simulink model "Backhoe_Arm"  (R2014a)
settings: Solver=ode23t  StartTime=0.0  StopTime=10  MaxStep=0.01  RelTol=1e-3
PostLoadFcn:
  | warning off sm:compiler:state:UnsatisfiedDesiredTarget
  | warning off simscape:compiler:sli:init:SolverNotRecommended
  | warning off sm:sli:visualization:UnsupportedSimMode
  | warning off xPCTarget:sampleTime:sampleTimeInvariance
  | warning off Simulink:blocks:MatchingFromNotFound
model workspace (MAT data in the model file):
  cylinderGray = [0.6 0.6 0.6]
  darkOrange = [0.8 0.5 0]
  glassBlue = [0.2 0.2 1]
  gray = [0.3 0.3 0.3]
  orange = [0.8 0.65 0]
  pistonGray = [0.4 0.4 0.4]
  tireBlack = [0.1 0.1 0.1]
  wheelGray = [0.6 0.6 0.6]
  yellow = [0.8 0.8 0]
  rhoGlass = 2500
  rhoRubber = 1500
  rhoSteel = 7800
undefined symbols (not defined in the file): sigbuilder_block, X, Y, Z
libraries: sm_lib x78, Backhoe_Lib x12, nesl_utility x3
(part 1 of 3)
Description:
  | Copyright 2014 The MathWorks, Inc.
settings Model: ExtModeTrigDuration=3334  BufferReuse=off  Creator=smiller  LastModifiedBy=Olli
settings SolverCC: EnableConcurrentExecution=on
settings DataIOCC: LimitDataPoints=off  SignalLoggingSaveFormat=ModelDataLogs
settings OptimizationCC: BlockReduction=off  OptimizeBlockIOStorage=off  BufferReuse=off  GlobalBufferReuse=off  ExpressionFolding=off  ExpressionDepthLimit=2147483647  LocalBlockOutputs=off
settings DebuggingCC: UnderspecifiedInitializationDetection=Classic  SolverPrmCheckMsg=none  MultiTaskDSMMsg=warning  MultiTaskCondExecSysMsg=none  StateNameClashWarn=warning
settings HardwareCC: ProdIntDivRoundTo=Zero  ProdEndianess=LittleEndian  ProdHWDeviceType=Generic->32-bit x86 compatible
settings RTWCC: SystemTargetFile=slrt.tlc  TemplateMakefile=slrt_default_tmf  Description=Simulink Real-Time  ProcessScript=slrt_make_rtw_hook  IncludeERTFirstTime=on  RTWCompilerOptimization=On
settings SimulinkRealTimeCC: GeneratePreprocessorConditionals=Disable all  EnableShiftOperators=on  RL32LogBufSizeModifier=300000
settings SimscapeCC: ExplicitSolverDiagnosticOptions=none
settings SimMechanicsCC: WarnOnRedundantConstraints=off
settings ExplorerConfigSet: InternalSimMechanicsExplorerSettings="<ExplorerConfiguration><canonicalview>default</canonicalview><TilePanel><TileInfo><Tiles Columns=\"1\" Count=\"1\" Rows=\"1\"><Column Left=\"2\" Weight=\"1\"/><Column Left=\"525\"/><Row Top=\"2\" Weight=\"1\"/><Row Top=\"370\"/><Tile Height=\"1\" Width=\"1\" X=\"0\" Y=\"0\"/></Tiles></TileInfo><SceneInfo><SceneViewer><BGColor><R>0.60000002384185791</R><G>0.60000002384185791</G><B>0.60000002384185791</B></BGColor><Camera><Position><X>16.211716622846833</X><Y>-13.061299378004865</Y><Z>8.3540336197668257</Z></Position><Center><X>-0.88618319905958465</X><Y>-6.5797450383619722</Y><Z>3.3077110306737345</Z></Center><Up><X>-0.26232421756367919</X><Y>0.057951672533943753</Y><Z>0.96323808507041631</Z></Up><Left>-4.3797052145004276</Left><Right>4.3797052145004276</Right><Bottom>-5.0912822484970093</Bottom><Top>5.0912822484970093</Top></Camera></SceneViewer></SceneInfo></TilePanel></ExplorerConfiguration>"

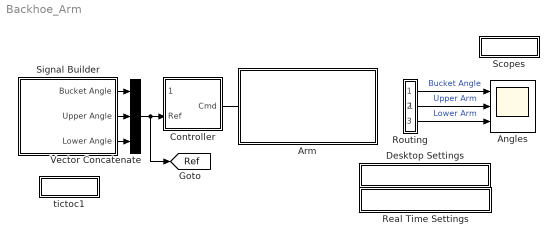
== system Backhoe_Arm ==
  Angles : Scope  NumInputPorts=3
      settings: TimeRange=60  YMin=-120~-20~-60  YMax=20~60~0
  Arm : Subsystem
      mask Display:
      | image(imread('Backhoe_Arm_IMAGE.JPG'));
      | port_label('input',1,'Cmd');
      | port_label('Output',1,'Meas');
  Controller : Subsystem
  Desktop Settings : Subsystem
      settings: OpenFcn=|
      | set_param(bdroot,'Solver','ODE23t','MaxStep','0.01','RelTol','1e-3','AbsTol','auto');
      | tvar_solverBlock = find_system(bdroot, 'SubClassName', 'solver');
      | 
      | for i=1:size(tvar_solverBlock,1)
      | 
      | set_param(char(tvar_solverBlock(i)), 'UseLocalSolver','off','DoFixedCost','off');
      | end
      | 
      | clear tvar_solverBlock
      mask Display: disp('Desktop Settings')
  Real Time Settings : Subsystem
      settings: OpenFcn=|
      | tvar_Nonlinear_Iterations = '2';
      | tvar_StepSize = '0.0004';                                                                                              %tvar_LocalSolver = 'NE_TRAPEZOIDAL_ADVANCER';
      | tvar_LocalSolver = 'NE_BACKWARD_EULER_ADVANCER';
      | set_param(bdroot,'Solver','ode1','FixedStep','auto');
      | tvar_solverBlock = find_system(bdroot, 'SubClassName', 'solver');
      | for i=1:size(tvar_solverBlock,1)
      | 
      | set_param(char(tvar_solverBlock(i)), 'UseLocalSolver','on','DoFixedCost','on','MaxNonlinIter',tvar_Nonlinear_Iterations,'LocalSolverChoice',tvar_LocalSolver,'LocalSolverSampleTime',tvar_StepSize);
      | end
      | clear tvar_Nonlinear_Iterations tvar_StepSize tvar_LocalSolver tvar_solverBlock
      mask Display: disp('Real Time Settings')
  Routing : Subsystem
  Scopes : Subsystem
  Signal Builder : Subsystem  Tag=STV Subsys  LoadFcn=sigbuilder_block('load');  StartFcn=sigbuilder_block('start');  StopFcn=sigbuilder_block('stop');  ClipboardFcn=sigbuilder_block('clipboard');  mask(Sigbuilder block){}
      mask help: Simulink:masks:SigbuilderBlock_MD
      mask init:
      | if ~strcmp(get_param(bdroot(gcbh),'SimulationStatus'),'stopped') tuvar = sigbuilder_block('maskInit'); end
      settings: CopyFcn=sigbuilder_block('copy');  DeleteFcn=sigbuilder_block('delete');  ModelCloseFcn=sigbuilder_block('modelClose');  PreSaveFcn=sigbuilder_block('preSave');  PauseFcn=sigbuilder_block('pause');  ContinueFcn=sigbuilder_block('continue');  NameChangeFcn=sigbuilder_block('namechange');  OpenFcn=sigbuilder_block('open',[5.58621 8.06897 624.414 412.759 ]);  CloseFcn=sigbuilder_block('close');
      mask Display: plot(0, 0, 100, 100,[2, 2, 32, 32, 2], [68, 8, 8, 68, 68],[32, 2], [38, 38], [32, 19, 2],[53, 60, 44], [32, 17, 17, 2],[16, 16, 31, 31]);txt = getActiveGroup(gcbh);text(2, 100, txt,'verticalAlignment', 'top');
  Vector Concatenate : Concatenate  NumInputs=3
  tictoc1 : Subsystem
      settings: OpenFcn=open('Backhoe_Demo_Script.html')
      mask Display: disp('Script')
  tag scope: Ref=global
  wires:
  Signal Builder/2(Upper Angle) -> Vector Concatenate/2
  Signal Builder/1(Bucket Angle) -> Vector Concatenate/1
  Signal Builder/3(Lower Angle) -> Vector Concatenate/3
  Vector Concatenate/1 -> [Ref], Controller/2(Ref)
  ? -> Controller/1(Meas), Routing/1(Meas)
  Controller/1(Cmd) -> ?
  Routing/2(UArm) -> Angles/2  "Upper Arm"
  Routing/3(LArm) -> Angles/3  "Lower Arm"
  Routing/1(Bucket) -> Angles/1  "Bucket Angle"

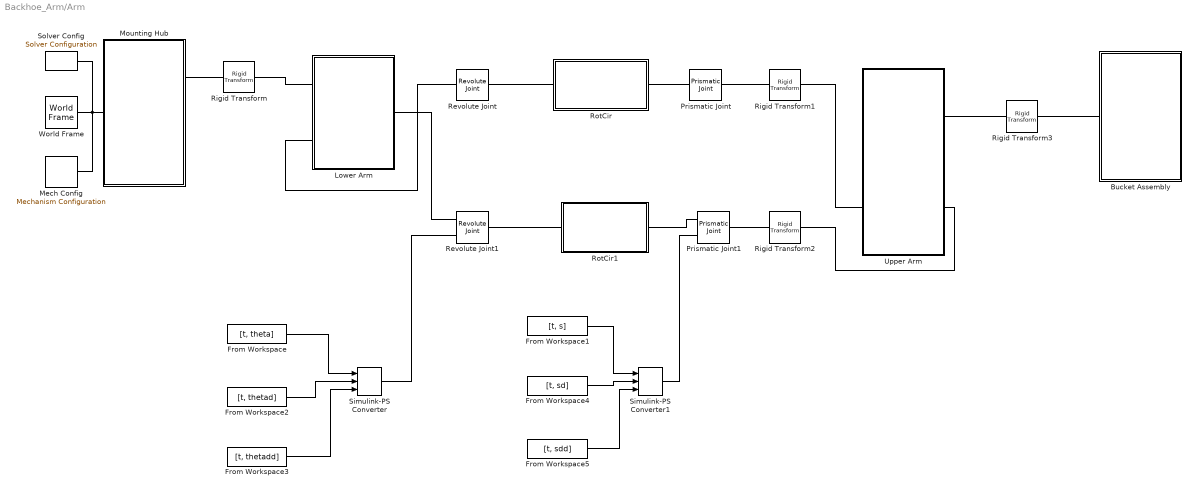
== system Backhoe_Arm/Arm ==
  Bucket Assembly : Subsystem
      mask Display:
      | image(imread('Backhoe_Arm_Bucket_Asy_IMAGE.JPG'));
      | port_label('lconn',1,'UAL');
      | port_label('lconn',2,'UAR');
      | port_label('lconn',3,'UA');
      | port_label('rconn',1,'TAct');
  From Workspace : FromWorkspace  VariableName=[t, theta]
  From Workspace1 : FromWorkspace  VariableName=[t, s]
  From Workspace2 : FromWorkspace  VariableName=[t, thetad]
  From Workspace3 : FromWorkspace  VariableName=[t, thetadd]
  From Workspace4 : FromWorkspace  VariableName=[t, sd]
  From Workspace5 : FromWorkspace  VariableName=[t, sdd]
  "Lower Arm " : Subsystem
      mask Display:
      | image(imread('Backhoe_Arm_Lower_IMAGE.JPG'));
      | port_label('lconn',1,'H');
      | port_label('lconn',2,'LAct');
      | port_label('rconn',1,'UA');
      | port_label('rconn',2,'RAct');
  Mech Config : sm_lib/Utilities/Mechanism Configuration  UniformGravity=Constant  GravityVector=[0 0 -9.81]  GravityUnits=m/s^2  LinearizationDelta=0.001  BlockFunction=simmechanics.library.utilities.mechanism_configuration
  Mounting Hub : Subsystem  mask(Mounting Hub){Hleft=1, Hright=2, Ltop=0.75, Lbottom=1.5, Tplate=0.3, Dplates=1.2, plateFillet=0.25, numPoints=15, L1=0.75, H1=0.25, RH1=0.075, L2=0.75, H2=1.75, RH2=0.075, L3=0.5, H3=0.5, Larm=0.8, Warm=0.5, Tarm=0.5, Tab=0.1, RH3=0.075, Dbracket=1.1, Lbracket=1.2, Wbracket=1.2, Tbracket=2, Hbracket=1, Rhole=0.1, Hhole=0.5, hubColor=orange, rho=rhoSteel}
      mask prompts: Hleft "Hleft [m]"; Hright "Hright [m]"; Ltop "Ltop [m]"; Lbottom "Lbottom [m]"; Tplate "Tplate [m]"; Dplates "Dplates [m]"; plateFillet "Plate Fillet Radius [m]"; numPoints "Fillet Point Resolution"; L1 "L1 [m]"; H1 "H1 [m]"; RH1 "RH1 [m]"; L2 "L2 [m]"; H2 "H2 [m]"; RH2 "RH2 [m]"; L3 "L3 [m]"; H3 "H3 [m]"; Larm "Larm [m]"; Warm "Warm [m]"; Tarm "Tarm [m]"; Tab "Tab [m]"; RH3 "RH3 [m]"; Dbracket "Dbracket [m]"; Lbracket "Lbracket [m]"; Wbracket "Wbracket [m]"; Tbracket "Tbracket [m]"; Hbracket "Hbracket [m]"; Rhole "Rhole [m]"; Hhole "Hhole [m]"; hubColor "Hub Color"; rho "Density [kg/m^3]"
      mask help:
      | Consists of the backhoe mounting hub assembly.
      |
      | This assembly connects to the Backhoe Arm assembly on the front end, and to the Mounting Base assembly on the rear and side.
      |
      | Attachment points are:
      | LH: Left base hydraulic actuator (piston Head).
      | RH: Right base hydraulic actuator (piston Head).
      | LC: Lower arm hydraulic actuator (Cylinder base).
      | LA: Lower Arm joint.
      | MB: Mounting Base joint.
      | All attachments are configured for Revolute Joints.
      |
      | Click on Help to view a schematic of the bracket, its configurable dimension parameters and attachment points (in red).
      mask init:
      | plateSection = [0              0     ; ...
      |                 Lbottom        0     ; ...
      |                 Lbottom        Hright; ...
      |                 (Lbottom-Ltop) Hright; ...
      |                 0              Hleft];
      | plateSection = Extr_Data_Round_Corners(plateSection,1:5,0.1,15);
      mask Help: web('Backhoe_Mountinghub.html');
      mask Display:
      | image(imread('Backhoe_Arm_Base_IMAGE.JPG'));
      | port_label('lconn',1,'B');
      | port_label('rconn',1,'LArm');
      | port_label('rconn',2,'LAct');
  Prismatic Joint : sm_lib/Joints/Prismatic Joint  SenseConstraintForce=off  SenseConstraintForceX=off  SenseConstraintForceY=off  SenseConstraintForceZ=off  SenseConstraintTorque=off  SenseConstraintTorqueX=off  SenseConstraintTorqueY=off  SenseConstraintTorqueZ=off  SenseTotalForce=off  SenseTotalForceX=off  SenseTotalForceY=off  SenseTotalForceZ=off  SenseTotalTorque=off  SenseTotalTorqueX=off  SenseTotalTorqueY=off  SenseTotalTorqueZ=off  CompositeWrenchDir=FollowerOnBase  CompositeWrenchFrame=BaseFrame  EquilibriumPosition=0  EquilibriumPositionUnits=m  SpringStiffness=0  SpringStiffnessUnits=N/m  DampingCoefficient=0  DampingCoefficientUnits=N/(m/s)  TorqueActuationMode=NoTorque  MotionActuationMode=ComputedMotion  SensePosition=off  SenseVelocity=off  SenseAcceleration=off  SenseTorqueForce=off  PositionTargetValue=0  PositionTargetValueUnits=m  PositionTargetSpecify=off  PositionTargetPriority=High  VelocityTargetValue=0.001  VelocityTargetValueUnits=m/s  VelocityTargetSpecify=on  VelocityTargetPriority=High  BlockFunction=simmechanics.library.joints.prismatic_joint
  Prismatic Joint1 : sm_lib/Joints/Prismatic Joint  SenseConstraintForce=off  SenseConstraintForceX=off  SenseConstraintForceY=off  SenseConstraintForceZ=off  SenseConstraintTorque=off  SenseConstraintTorqueX=off  SenseConstraintTorqueY=off  SenseConstraintTorqueZ=off  SenseTotalForce=off  SenseTotalForceX=off  SenseTotalForceY=off  SenseTotalForceZ=off  SenseTotalTorque=off  SenseTotalTorqueX=off  SenseTotalTorqueY=off  SenseTotalTorqueZ=off  CompositeWrenchDir=FollowerOnBase  CompositeWrenchFrame=BaseFrame  EquilibriumPosition=0  EquilibriumPositionUnits=m  SpringStiffness=0  SpringStiffnessUnits=N/m  DampingCoefficient=0  DampingCoefficientUnits=N/(m/s)  TorqueActuationMode=ComputedTorque  MotionActuationMode=InputMotion  SensePosition=off  SenseVelocity=off  SenseAcceleration=off  SenseTorqueForce=off  PositionTargetValue=0  PositionTargetValueUnits=m  PositionTargetSpecify=off  PositionTargetPriority=High  VelocityTargetValue=0.001  VelocityTargetValueUnits=m/s  VelocityTargetSpecify=on  VelocityTargetPriority=High  BlockFunction=simmechanics.library.joints.prismatic_joint
  Revolute Joint : sm_lib/Joints/Revolute Joint  SenseConstraintForce=off  SenseConstraintForceX=off  SenseConstraintForceY=off  SenseConstraintForceZ=off  SenseConstraintTorque=off  SenseConstraintTorqueX=off  SenseConstraintTorqueY=off  SenseConstraintTorqueZ=off  SenseTotalForce=off  SenseTotalForceX=off  SenseTotalForceY=off  SenseTotalForceZ=off  SenseTotalTorque=off  SenseTotalTorqueX=off  SenseTotalTorqueY=off  SenseTotalTorqueZ=off  CompositeWrenchDir=FollowerOnBase  CompositeWrenchFrame=BaseFrame  EquilibriumPosition=0  EquilibriumPositionUnits=deg  SpringStiffness=0  SpringStiffnessUnits=N*m/deg  DampingCoefficient=0  DampingCoefficientUnits=N*m/(deg/s)  TorqueActuationMode=NoTorque  MotionActuationMode=ComputedMotion  SensePosition=off  SenseVelocity=off  SenseAcceleration=off  SenseTorqueForce=off  PositionTargetValue=0  PositionTargetValueUnits=deg  PositionTargetSpecify=off  PositionTargetPriority=High  VelocityTargetValue=45  VelocityTargetValueUnits=deg/s  VelocityTargetSpecify=off  VelocityTargetPriority=High  BlockFunction=simmechanics.library.joints.revolute_joint
  Revolute Joint1 : sm_lib/Joints/Revolute Joint  SenseConstraintForce=off  SenseConstraintForceX=off  SenseConstraintForceY=off  SenseConstraintForceZ=off  SenseConstraintTorque=off  SenseConstraintTorqueX=off  SenseConstraintTorqueY=off  SenseConstraintTorqueZ=off  SenseTotalForce=off  SenseTotalForceX=off  SenseTotalForceY=off  SenseTotalForceZ=off  SenseTotalTorque=off  SenseTotalTorqueX=off  SenseTotalTorqueY=off  SenseTotalTorqueZ=off  CompositeWrenchDir=FollowerOnBase  CompositeWrenchFrame=BaseFrame  EquilibriumPosition=0  EquilibriumPositionUnits=deg  SpringStiffness=0  SpringStiffnessUnits=N*m/deg  DampingCoefficient=0  DampingCoefficientUnits=N*m/(deg/s)  TorqueActuationMode=ComputedTorque  MotionActuationMode=InputMotion  SensePosition=off  SenseVelocity=off  SenseAcceleration=off  SenseTorqueForce=off  PositionTargetValue=0  PositionTargetValueUnits=deg  PositionTargetSpecify=off  PositionTargetPriority=High  VelocityTargetValue=45  VelocityTargetValueUnits=deg/s  VelocityTargetSpecify=off  VelocityTargetPriority=High  BlockFunction=simmechanics.library.joints.revolute_joint
  Rigid Transform : sm_lib/Frames and Transforms/Rigid Transform  TranslationMethod=None  TranslationLengthUnit=m  TranslationStandardAxis=+Z  TranslationStandardOffset=0  TranslationCartesianOffset=[0 0 0]  TranslationROffset=0  TranslationROffsetUnits=m  TranslationZOffset=0  TranslationZOffsetUnits=m  TranslationThetaOffset=0  TranslationThetaOffsetUnits=deg  RotationMethod=StandardAxis  RotationAngleUnits=rad  RotationStandardAxis=-Z  RotationAngle=pi/4  RotationArbitraryAxis=[0 0 1]  FollAlignAxisA=+X  BaseAlignAxisA=+Y  FollAlignAxisB=+Y  BaseAlignAxisB=+Z  BlockFunction=simmechanics.library.frames_transforms.rigid_transform
  Rigid Transform1 : sm_lib/Frames and Transforms/Rigid Transform  TranslationMethod=None  TranslationLengthUnit=m  TranslationStandardAxis=+Z  TranslationStandardOffset=0  TranslationCartesianOffset=[0 0 0]  TranslationROffset=0  TranslationROffsetUnits=m  TranslationZOffset=0  TranslationZOffsetUnits=m  TranslationThetaOffset=0  TranslationThetaOffsetUnits=deg  RotationMethod=AlignedAxes  RotationAngleUnits=deg  RotationStandardAxis=-Z  RotationAngle=50  RotationArbitraryAxis=[0 0 1]  FollAlignAxisA=+Z  BaseAlignAxisA=+Z  FollAlignAxisB=+Y  BaseAlignAxisB=-X  BlockFunction=simmechanics.library.frames_transforms.rigid_transform
  Rigid Transform2 : sm_lib/Frames and Transforms/Rigid Transform  TranslationMethod=None  TranslationLengthUnit=m  TranslationStandardAxis=+Z  TranslationStandardOffset=0  TranslationCartesianOffset=[0 0 0]  TranslationROffset=0  TranslationROffsetUnits=m  TranslationZOffset=0  TranslationZOffsetUnits=m  TranslationThetaOffset=0  TranslationThetaOffsetUnits=deg  RotationMethod=AlignedAxes  RotationAngleUnits=deg  RotationStandardAxis=-Z  RotationAngle=50  RotationArbitraryAxis=[0 0 1]  FollAlignAxisA=+Z  BaseAlignAxisA=+Z  FollAlignAxisB=+Y  BaseAlignAxisB=-X  BlockFunction=simmechanics.library.frames_transforms.rigid_transform
  Rigid Transform3 : sm_lib/Frames and Transforms/Rigid Transform  TranslationMethod=None  TranslationLengthUnit=m  TranslationStandardAxis=+Z  TranslationStandardOffset=0  TranslationCartesianOffset=[0 0 0]  TranslationROffset=0  TranslationROffsetUnits=m  TranslationZOffset=0  TranslationZOffsetUnits=m  TranslationThetaOffset=0  TranslationThetaOffsetUnits=deg  RotationMethod=StandardAxis  RotationAngleUnits=deg  RotationStandardAxis=-Z  RotationAngle=90  RotationArbitraryAxis=[0 0 1]  FollAlignAxisA=+X  BaseAlignAxisA=+Y  FollAlignAxisB=+Y  BaseAlignAxisB=+Z  BlockFunction=simmechanics.library.frames_transforms.rigid_transform
  "RotCir " : Subsystem
  RotCir1 : Subsystem
  Simulink-PS Converter : nesl_utility/Simulink-PS Converter  PhysicalDomain=network_engine_domain  SubClassName=ps_input  LeftPortType=input  RightPortType=output  PseudoPeriodic=off  Frequencies=[]  NoiseDistribution=none  NoiseParameters=[]  Unit=1  AffineConversion=off  InputFiltering=derivs  SimscapeFilterOrder=1  InputFilterTimeConstant=0.001  UdotUserProvided=2
  Simulink-PS Converter1 : nesl_utility/Simulink-PS Converter  PhysicalDomain=network_engine_domain  SubClassName=ps_input  LeftPortType=input  RightPortType=output  PseudoPeriodic=off  Frequencies=[]  NoiseDistribution=none  NoiseParameters=[]  Unit=1  AffineConversion=off  InputFiltering=derivs  SimscapeFilterOrder=1  InputFilterTimeConstant=0.001  UdotUserProvided=2
  Solver Config : nesl_utility/Solver Configuration  PhysicalDomain=network_engine_domain  SubClassName=solver  LeftPortType=input  RightPortType=generic  Accelerate=off  Tones=[]  Harmonics=[]  SimulateNoise=off  Profile=off  UseLocalSampling=off  EnableSwitchedLinearOptims=on  FrequencyDomain=off  UseCCode=off  RelTol=0.001  AbsTol=1e-06  MinStep=1e-09  ToWorkspace=off  DoDC=off  ResidualTolerance=1e-9  UseLocalSolver=off  LocalSolverChoice=NE_BACKWARD_EULER_ADVANCER  LocalSolverSampleTime=0.0004  DoFixedCost=off  MaxNonlinIter=2  MaxModeIter=2  LinearAlgebra=Sparse  DelaysMemoryBudget=1024  AutomaticFiltering=on  FilteringTimeConstant=0.001
  Upper Arm : Subsystem
      mask Display:
      | image(imread('Backhoe_Arm_Upper_IMAGE.JPG'));
      | port_label('lconn',1,'LA');
      | port_label('lconn',2,'RAct');
      | port_label('rconn',1,'CrL');
      | port_label('rconn',2,'CrR');
      | port_label('rconn',3,'B');
      | port_label('rconn',4,'TAct');
  World Frame : sm_lib/Frames and Transforms/World Frame  BlockFunction=simmechanics.library.frames_transforms.world_frame
  wires:
  From Workspace/1 -> Simulink-PS Converter/1
  From Workspace2/1 -> Simulink-PS Converter/2
  From Workspace3/1 -> Simulink-PS Converter/3
  From Workspace1/1 -> Simulink-PS Converter1/1
  From Workspace4/1 -> Simulink-PS Converter1/2
  From Workspace5/1 -> Simulink-PS Converter1/3
  connections:
  Mech Config/RConn1 -- Mounting Hub/LConn1 -- Solver Config/RConn1 -- World Frame/RConn1
  Rigid Transform/LConn1 -- Mounting Hub/RConn1
  Rigid Transform/RConn1 -- "Lower Arm "/LConn1
  Revolute Joint/RConn1 -- "RotCir "/LConn1
  Revolute Joint1/RConn1 -- RotCir1/LConn1
  Rigid Transform2/RConn1 -- Upper Arm/RConn2
  Rigid Transform1/RConn1 -- Upper Arm/LConn2
  Revolute Joint/LConn1 -- "Lower Arm "/LConn2
  "Lower Arm "/RConn1 -- Revolute Joint1/LConn1
  Rigid Transform3/LConn1 -- Upper Arm/RConn1
  Rigid Transform3/RConn1 -- Bucket Assembly/LConn1
  Prismatic Joint/RConn1 -- Rigid Transform1/LConn1
  Prismatic Joint/LConn1 -- "RotCir "/RConn1
  Prismatic Joint1/LConn1 -- RotCir1/RConn1
  Prismatic Joint1/RConn1 -- Rigid Transform2/LConn1
  Simulink-PS Converter/RConn1 -- Revolute Joint1/LConn2
  Simulink-PS Converter1/RConn1 -- Prismatic Joint1/LConn2

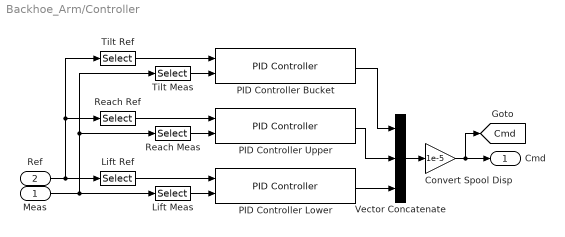
== system Backhoe_Arm/Controller ==
  Meas : Inport
  Ref : Inport  Port=2
  Convert Spool Disp : Gain  Gain=1e-5
  Lift Meas : Selector  InputPortWidth=3  Indices=3
  Lift Ref : Selector  InputPortWidth=3  Indices=3
  PID Controller Bucket : Backhoe_Lib/PID Controller  upperLim=10  lowerLim=-120  Kp=10  Ki=0.01  Kd=0.01  N=100
  PID Controller Lower : Backhoe_Lib/PID Controller  upperLim=40  lowerLim=-70  Kp=30  Ki=0.002  Kd=0.002  N=100
  PID Controller Upper : Backhoe_Lib/PID Controller  upperLim=60  lowerLim=-20  Kp=24  Ki=0  Kd=0  N=100
  Reach Meas : Selector  InputPortWidth=3  Indices=2
  Reach Ref : Selector  InputPortWidth=3  Indices=2
  "Tilt Meas " : Selector  InputPortWidth=3
  Tilt Ref : Selector  InputPortWidth=3
  Vector Concatenate : Concatenate  NumInputs=3
  Cmd : Outport
  tag scope: Cmd=global
  wires:
  "Tilt Meas "/1 -> PID Controller Bucket/2
  Tilt Ref/1 -> PID Controller Bucket/1
  Reach Meas/1 -> PID Controller Upper/2
  Reach Ref/1 -> PID Controller Upper/1
  Lift Ref/1 -> PID Controller Lower/1
  Lift Meas/1 -> PID Controller Lower/2
  Meas/1 -> "Tilt Meas "/1, Reach Meas/1, Lift Meas/1
  Ref/1 -> Lift Ref/1, Tilt Ref/1, Reach Ref/1
  Vector Concatenate/1 -> Convert Spool Disp/1
  Convert Spool Disp/1 -> Cmd/1, [Cmd]
  PID Controller Upper/1 -> Vector Concatenate/2
  PID Controller Lower/1 -> Vector Concatenate/3
  PID Controller Bucket/1 -> Vector Concatenate/1

== system Backhoe_Arm/Desktop Settings ==

== system Backhoe_Arm/Real Time Settings ==

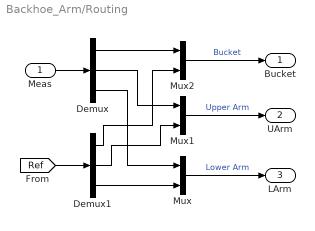
== system Backhoe_Arm/Routing ==
  Meas : Inport
  Demux : Demux  Outputs=3
  Demux1 : Demux  Outputs=3
  Mux : Mux  Inputs=2
  Mux1 : Mux  Inputs=2
  Mux2 : Mux  Inputs=2
  Bucket : Outport
  UArm : Outport  Port=2
  LArm : Outport  Port=3
  wires:
  Demux/3 -> Mux/1
  Demux/2 -> Mux1/1
  Demux1/1 -> Mux2/2
  Mux/1 -> LArm/1  "Lower Arm"
  Mux1/1 -> UArm/1  "Upper Arm"
  Demux/1 -> Mux2/1
  Demux1/3 -> Mux/2
  Demux1/2 -> Mux1/2
  Mux2/1 -> Bucket/1  "Bucket"
  [Ref] -> Demux1/1
  Meas/1 -> Demux/1

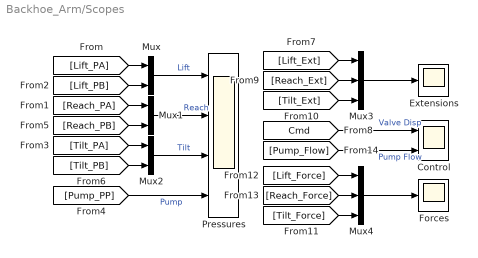
== system Backhoe_Arm/Scopes ==
  Control : Scope  NumInputPorts=2
      settings: TimeRange=60  YMin=-0.01~5200  YMax=0.01~5220
  Extensions : Scope
      settings: TimeRange=60  YMin=0  YMax=2.5  SaveName=ScopeData2
  Forces : Scope
      settings: TimeRange=60  YMin=-8000000  YMax=2000000  SaveName=ScopeData3
  Mux : Mux  Inputs=2
  Mux1 : Mux  Inputs=2
  Mux2 : Mux  Inputs=2
  Mux3 : Mux  Inputs=3
  Mux4 : Mux  Inputs=3
  Pressures : Scope  NumInputPorts=4
      settings: TimeRange=60  YMin=0~0~8000000~27600000  YMax=30000000~25000000~20000000~28400000  SaveName=Cyl_Press_DATA
  wires:
  [Pump_PP] -> Pressures/4  "Pump"
  Mux/1 -> Pressures/1  "Lift"
  [Lift_PA] -> Mux/1
  [Lift_PB] -> Mux/2
  [Reach_PA] -> Mux1/1
  Mux1/1 -> Pressures/2  "Reach"
  [Reach_PB] -> Mux1/2
  [Tilt_PA] -> Mux2/1
  Mux2/1 -> Pressures/3  "Tilt"
  [Tilt_PB] -> Mux2/2
  [Lift_Ext] -> Mux3/1
  [Reach_Ext] -> Mux3/2
  [Tilt_Ext] -> Mux3/3
  Mux3/1 -> Extensions/1
  [Cmd] -> Control/1  "Valve Disp"
  [Lift_Force] -> Mux4/1
  [Reach_Force] -> Mux4/2
  [Tilt_Force] -> Mux4/3
  Mux4/1 -> Forces/1
  [Pump_Flow] -> Control/2  "Pump Flow"

== system Backhoe_Arm/Signal Builder ==
  Demux : Demux  Tag=STV Demux  Outputs=3
  FromWs : FromWorkspace  Tag=STV FromWs  VariableName=tuvar  SampleTime=0  OutputAfterFinalValue=Holding final value
      SigBuilderData=|
      | common.afterFinalStr = 'Hold final value'
      | common.sampleTime = '0'
      | dataSet.timeRange = [0 60]
      | dataSet.name = 'Ref'
      | sbobj.Groups.Name = 'Ref'
      | sbobj.Groups.Signals(1).Name = 'Bucket Angle'
      | sbobj.Groups.Signals(1).XData = [0 7 11 24 28.5 40 43 51.5 53.5 60]
      | sbobj.Groups.Signals(1).YData = [0 0 -90 -90 0 0 -110 -110 0 0]
      | sbobj.Groups.Signals(2).Name = 'Upper Angle'
      | sbobj.Groups.Signals(2).XData = [0 12.5 25 30 32.5 54 60]
      | sbobj.Groups.Signals(2).YData = [50 50 -20 -20 40 55 55]
      | sbobj.Groups.Signals(3).Name = 'Lower Angle'
      | sbobj.Groups.Signals(3).XData = [0 15 27.5 30 40 60]
      | sbobj.Groups.Signals(3).YData = [-60 -60 -30 -30 -60 -60]
      | sbobj.Groups.TimeRange = [0 60]
  Bucket Angle : Outport  Tag=STV Outport
  Upper Angle : Outport  Tag=STV Outport  Port=2
  Lower Angle : Outport  Tag=STV Outport  Port=3
  wires:
  Demux/3 -> Lower Angle/1
  Demux/2 -> Upper Angle/1
  FromWs/1 -> Demux/1
  Demux/1 -> Bucket Angle/1

== system Backhoe_Arm/tictoc1 ==

== system Backhoe_Arm/Arm/Bucket Assembly ==
  Bucket : Subsystem  mask(Bucket){plateSide=1.2, plateFilletR=0.2, plateDist=1.2, plateWidth=0.2, plateHoleR=0.075, bucketHeight=2, bucketLength=2, bucketThickness=0.05, bucketUpper=1.3, bucketLower=2, chordAngle=pi/6, toothLength=0.25, toothWidth=0.2, toothTip=0.025, circlePoints=45, bucketColor=yellow, bracketColor=yellow, rho=rhoSteel}
      mask prompts: plateSide "Wplate [m]"; plateFilletR "Rfillet [m]"; plateDist "Dplate [m]"; plateWidth "Tplate [m]"; plateHoleR "Rpin [m]"; bucketHeight "Hbucket [m]"; bucketLength "Wbucket [m]"; bucketThickness "Tbucket [m]"; bucketUpper "Wupper [m]"; bucketLower "Wlower [m]"; chordAngle "alpha [radians]"; toothLength "Ltooth [m]"; toothWidth "Wtooth [m]"; toothTip "Ttooth [m]"; circlePoints "Circle Mesh Resolution"; bucketColor "Bucket Color"; bracketColor "Bracket Color"; rho "Density [kg/m^3]"
      mask help:
      | Consists of the backhoe bucket assembly with attachment frame.
      |
      | Attachment points are:
      | CA: Center point of the Crank Arm link pin.
      | UA: Center Point of the Upper Arm link pin.
      | Both points are configured for Revolute joints.
      |
      | Click on Help to view a schematic of the bucket, its configurable dimension parameters and attachment points (in red).
      mask init:
      | bucketRadius = bucketHeight/(2*cos(chordAngle));
      | 
      | % Bucket Back
      | bucketBack = [];
      | % Outer wall
      | for i = 0:circlePoints;
      |    angle = (-pi/2+chordAngle) + (pi - 2*chordAngle)*(i/circlePoints);
      |    bucketBack = [bucketBack; ...
      |        (bucketRadius*cos(angle)-bucketRadius*sin(chordAngle)) ...
      |         bucketRadius*sin(angle)];
      | end
      | 
      | % Inner Wall
      | beta = acos( ( (bucketRadius*cos(chordAngle) - bucketThickness/cos(chordAngle)) ...
      |                    /(bucketRadius-bucketThickness)) );
      | for i = 0:circlePoints;
      |    angle = (pi/2 - beta) - (pi-2*beta)*(i/circlePoints);
      |    bucketBack = [bucketBack; ...
      |        ((bucketRadius-bucketThickness)*cos(angle)-bucketRadius*sin(chordAngle)) ... 
      |        (bucketRadius-bucketThickness)*sin(angle)];
      | end
      | 
      | bucketBack = [bucketBack; ...
      |               -bucketLower -(bucketHeight/2-bucketThickness);...
      |               -bucketLower -bucketHeight/2];
      |           
      | % Uncomment below to plot the cross-sections. 
      | % close all
      | % figure
      | % plot(bucketBack(:,1),bucketBack(:,2));
      mask Help: web('Backhoe_Bucket.html');
      mask Display:
      | image(imread('Backhoe_Bucket_IMAGE.png'));
      | port_label('rconn',1,'CA');
      | port_label('rconn',2,'UA');
  UA : PMIOPort  Port=1  Side=Left
  connections:
  Bucket/RConn1 -- UA/RConn1

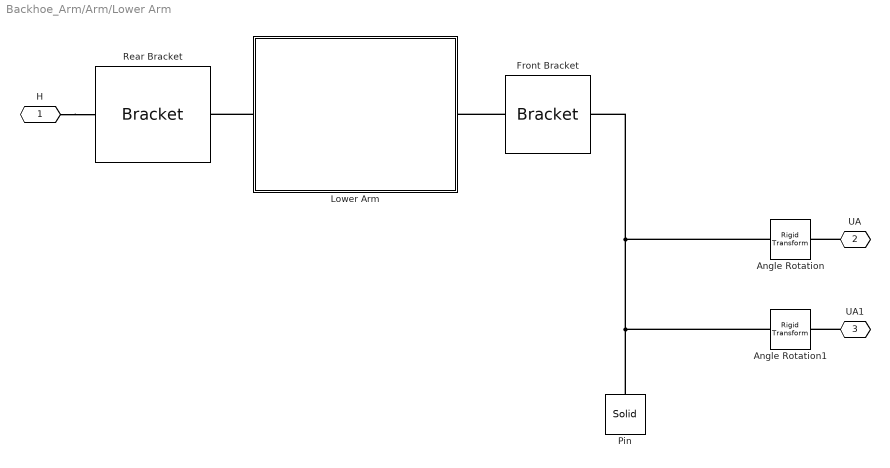
== system Backhoe_Arm/Arm/Lower Arm  ==
  Angle Rotation : sm_lib/Frames and Transforms/Rigid Transform  TranslationMethod=StandardAxis  TranslationLengthUnit=m  TranslationStandardAxis=+Z  TranslationStandardOffset=0.5  TranslationCartesianOffset=[0 0 0]  TranslationROffset=0  TranslationROffsetUnits=m  TranslationZOffset=0  TranslationZOffsetUnits=m  TranslationThetaOffset=0  TranslationThetaOffsetUnits=deg  RotationMethod=AlignedAxes  RotationAngleUnits=deg  RotationStandardAxis=+Z  RotationAngle=180  RotationArbitraryAxis=[0 0 1]  FollAlignAxisA=+Z  BaseAlignAxisA=+Z  FollAlignAxisB=+Y  BaseAlignAxisB=-Y  BlockFunction=simmechanics.library.frames_transforms.rigid_transform
  Angle Rotation1 : sm_lib/Frames and Transforms/Rigid Transform  TranslationMethod=StandardAxis  TranslationLengthUnit=m  TranslationStandardAxis=-Z  TranslationStandardOffset=0.5  TranslationCartesianOffset=[0 0 0]  TranslationROffset=0  TranslationROffsetUnits=m  TranslationZOffset=0  TranslationZOffsetUnits=m  TranslationThetaOffset=0  TranslationThetaOffsetUnits=deg  RotationMethod=AlignedAxes  RotationAngleUnits=deg  RotationStandardAxis=+Z  RotationAngle=180  RotationArbitraryAxis=[0 0 1]  FollAlignAxisA=+Z  BaseAlignAxisA=+Z  FollAlignAxisB=+Y  BaseAlignAxisB=-Y  BlockFunction=simmechanics.library.frames_transforms.rigid_transform
  Front Bracket : Backhoe_Lib/Bracket  Hbracket=5  Wbracket=0.8  Tbracket=0.65  Dbracket=0.45  Hhole=0.4  Rhole=0.075  circlePoints=25  bracketColor=yellow  rho=rhoSteel
  Lower Arm : Subsystem  mask(Lower Arm){Lbar=9, Wbar=0.8, Tbar=0.85, Lb=0.5, barFillet=0.1, numPoints=15, armColor=yellow, rho=rhoSteel}
      mask prompts: Lbar "Lbar [m]"; Wbar "Wbar [m]"; Tbar "Tbar [m]"; Lb "Lb [m]"; barFillet "Bar Fillet Radius [m]"; numPoints "Fillet Point Resolution"; armColor "Arm Color"; rho "Density [kg/m^3]"
      mask help:
      | Consists of the backhoe lower arm and three attachment brackets -- front, rear and upper
      |
      | Attachment Points are:
      | MA: Mounting Assembly attachment.
      | LH: Lower arm hydraulic actuator (piston Head).
      | UA: Upper arm attachment.
      | UC: Upper arm hydraulic actuator (Cylinder base).
      | All attachments are configured for Revolute joints.
      |
      | The length Lb corresponds to the lengths measured from the center of the bar to the center of the upper bracket.
      |
      | The front and rear brackets are automatically placed at the center of the end faces of the upper arm bar.
      |
      | Click on Help to view a schematic of the lower arm, its configurable dimension parameters and attachment points (in red).
      mask init:
      | barSection = [Tbar/2 Wbar/2;  ...
      |              -Tbar/2 Wbar/2;  ...
      |              -Tbar/2 -Wbar/2; ...
      |               Tbar/2 -Wbar/2];
      | barSection = Extr_Data_Round_Corners(barSection,1:4,barFillet,numPoints);
      mask Help: web('Backhoe_lowerarm.html');
      mask Display:
      | image(imread('Backhoe_Lowerarm_IMAGE.png'));
      | port_label('rconn',1,'RB');
      | port_label('lconn',2,'FB');;
      | port_label('lconn',1,'UB');
  Pin : sm_lib/Body Elements/Solid  InertiaType=CalculateFromGeometry  Mass=1  MassUnits=kg  CenterOfMass=[0 0 0]  CenterOfMassUnits=m  MomentsOfInertia=[1 1 1]  MomentsOfInertiaUnits=kg*m^2  ProductsOfInertia=[0 0 0]  ProductsOfInertiaUnits=kg*m^2  DensityBased=on  Density=rhoSteel  DensityUnits=kg/(m^3)  GraphicType=FromGeometry  MarkerShape=Sphere  MarkerSize=10  MarkerSizeUnits=m  GraphicVisPropType=SimpleVisualProperties  GraphicDiffuseColor=gray  GraphicSpecularColor=[0.5 0.5 0.5 1.0]  GraphicAmbientColor=[0.15 0.15 0.15 1.0]  GraphicEmissiveColor=[0.0 0.0 0.0 1.0]  GraphicShininess=75  GraphicOpacity=1.0  GeometryShape=Cylinder  RectangleSize=[1 1]  RectangleSizeUnits=m  BrickDimensions=[1 1 1]  BrickDimensionUnits=m  CylinderRadius=0.075  CylinderRadiusUnits=m  CylinderLength=1.1  CylinderLengthUnits=m  SphereRadius=1  SphereRadiusUnits=m  EllipsoidRadii=[1 1 1]  EllipsoidRadiiUnits=m  ExtrusionCrossSection=[1 1; -1 1; -1 -1; 1 -1]  ExtrusionCrossSectionUnits=m  ExtrusionLength=1  ExtrusionLengthUnits=m  PolygonNumSides=3  PolygonOuterRadius=1  PolygonOuterRadiusUnits=m  ExtGeomFileType=STL  ExtGeomFileUnits=m  RevolutionCrossSection=[1 1; 1 -1; 2 -1; 2 1]  RevolutionCrossSectionUnits=m  RevolutionExtent=Full  RevolutionAngle=180  RevolutionAngleUnits=deg  BlockFunction=simmechanics.library.body_elements.solid
  Rear Bracket : Backhoe_Lib/Bracket  Hbracket=0.75  Wbracket=0.75  Tbracket=0.15  Dbracket=0.75  Hhole=0.5  Rhole=0.075  circlePoints=25  bracketColor=yellow  rho=rhoSteel
  H : PMIOPort  Port=1  Side=Left
  UA : PMIOPort  Port=2  Side=Right
  UA1 : PMIOPort  Port=3  Side=Left
  connections:
  H/RConn1 -- Rear Bracket/RConn1
  Lower Arm/RConn1 -- Rear Bracket/LConn1
  Pin/RConn1 -- Angle Rotation1/LConn1 -- Front Bracket/RConn1 -- Angle Rotation/LConn1
  Front Bracket/LConn1 -- Lower Arm/LConn1
  UA/RConn1 -- Angle Rotation/RConn1
  UA1/RConn1 -- Angle Rotation1/RConn1

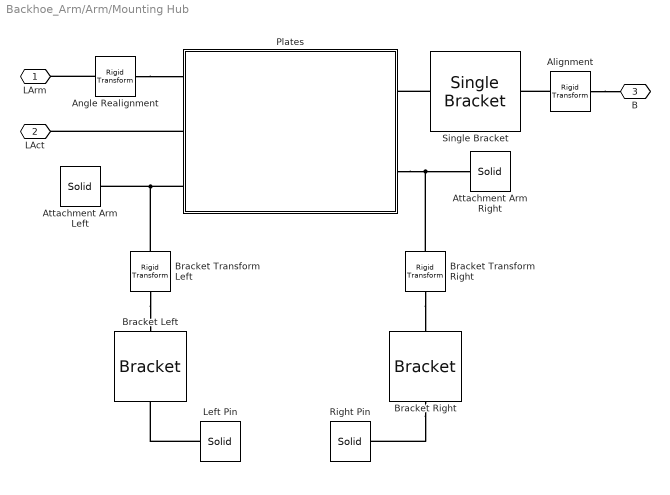
== system Backhoe_Arm/Arm/Mounting Hub ==
  Alignment : sm_lib/Frames and Transforms/Rigid Transform  TranslationMethod=None  TranslationLengthUnit=m  TranslationStandardAxis=+Z  TranslationStandardOffset=0  TranslationCartesianOffset=[0 0 0]  TranslationROffset=0  TranslationROffsetUnits=m  TranslationZOffset=0  TranslationZOffsetUnits=m  TranslationThetaOffset=0  TranslationThetaOffsetUnits=deg  RotationMethod=StandardAxis  RotationAngleUnits=deg  RotationStandardAxis=+Y  RotationAngle=180  RotationArbitraryAxis=[0 0 1]  FollAlignAxisA=+X  BaseAlignAxisA=+X  FollAlignAxisB=+Y  BaseAlignAxisB=+Z  BlockFunction=simmechanics.library.frames_transforms.rigid_transform
  Angle Realignment : sm_lib/Frames and Transforms/Rigid Transform  TranslationMethod=None  TranslationLengthUnit=m  TranslationStandardAxis=+Z  TranslationStandardOffset=0.5  TranslationCartesianOffset=[ 0 0 0]  TranslationROffset=0  TranslationROffsetUnits=m  TranslationZOffset=0  TranslationZOffsetUnits=m  TranslationThetaOffset=0  TranslationThetaOffsetUnits=deg  RotationMethod=AlignedAxes  RotationAngleUnits=deg  RotationStandardAxis=-Z  RotationAngle=90  RotationArbitraryAxis=[0 0 1]  FollAlignAxisA=+Z  BaseAlignAxisA=+Z  FollAlignAxisB=+X  BaseAlignAxisB=-Y  BlockFunction=simmechanics.library.frames_transforms.rigid_transform
  Attachment Arm Left : sm_lib/Body Elements/Solid  InertiaType=CalculateFromGeometry  Mass=1  MassUnits=kg  CenterOfMass=[0 0 0]  CenterOfMassUnits=m  MomentsOfInertia=[1 1 1]  MomentsOfInertiaUnits=kg*m^2  ProductsOfInertia=[0 0 0]  ProductsOfInertiaUnits=kg*m^2  DensityBased=on  Density=rho  DensityUnits=kg/(m^3)  GraphicType=FromGeometry  MarkerShape=Sphere  MarkerSize=10  MarkerSizeUnits=m  GraphicVisPropType=SimpleVisualProperties  GraphicDiffuseColor=hubColor  GraphicSpecularColor=[0.5 0.5 0.5 1.0]  GraphicAmbientColor=[0.15 0.15 0.15 1.0]  GraphicEmissiveColor=[0.0 0.0 0.0 1.0]  GraphicShininess=75  GraphicOpacity=1.0  GeometryShape=Brick  RectangleSize=[1 1]  RectangleSizeUnits=m  BrickDimensions=[Warm Tarm (Larm-Warm)]  BrickDimensionUnits=m  CylinderRadius=1  CylinderRadiusUnits=m  CylinderLength=1  CylinderLengthUnits=m  SphereRadius=1  SphereRadiusUnits=m  EllipsoidRadii=[1 1 1]  EllipsoidRadiiUnits=m  ExtrusionCrossSection=plateSection  ExtrusionCrossSectionUnits=m  ExtrusionLength=Tplate  ExtrusionLengthUnits=m  PolygonNumSides=3  PolygonOuterRadius=1  PolygonOuterRadiusUnits=m  ExtGeomFileType=STL  ExtGeomFileUnits=m  RevolutionCrossSection=[1 1; 1 -1; 2 -1; 2 1]  RevolutionCrossSectionUnits=m  RevolutionExtent=Full  RevolutionAngle=180  RevolutionAngleUnits=deg  BlockFunction=simmechanics.library.body_elements.solid
  Attachment Arm Right : sm_lib/Body Elements/Solid  InertiaType=CalculateFromGeometry  Mass=1  MassUnits=kg  CenterOfMass=[0 0 0]  CenterOfMassUnits=m  MomentsOfInertia=[1 1 1]  MomentsOfInertiaUnits=kg*m^2  ProductsOfInertia=[0 0 0]  ProductsOfInertiaUnits=kg*m^2  DensityBased=on  Density=rho  DensityUnits=kg/(m^3)  GraphicType=FromGeometry  MarkerShape=Sphere  MarkerSize=10  MarkerSizeUnits=m  GraphicVisPropType=SimpleVisualProperties  GraphicDiffuseColor=hubColor  GraphicSpecularColor=[0.5 0.5 0.5 1.0]  GraphicAmbientColor=[0.15 0.15 0.15 1.0]  GraphicEmissiveColor=[0.0 0.0 0.0 1.0]  GraphicShininess=75  GraphicOpacity=1.0  GeometryShape=Brick  RectangleSize=[1 1]  RectangleSizeUnits=m  BrickDimensions=[Warm Tarm (Larm-Warm)]  BrickDimensionUnits=m  CylinderRadius=1  CylinderRadiusUnits=m  CylinderLength=1  CylinderLengthUnits=m  SphereRadius=1  SphereRadiusUnits=m  EllipsoidRadii=[1 1 1]  EllipsoidRadiiUnits=m  ExtrusionCrossSection=plateSection  ExtrusionCrossSectionUnits=m  ExtrusionLength=Tplate  ExtrusionLengthUnits=m  PolygonNumSides=3  PolygonOuterRadius=1  PolygonOuterRadiusUnits=m  ExtGeomFileType=STL  ExtGeomFileUnits=m  RevolutionCrossSection=[1 1; 1 -1; 2 -1; 2 1]  RevolutionCrossSectionUnits=m  RevolutionExtent=Full  RevolutionAngle=180  RevolutionAngleUnits=deg  BlockFunction=simmechanics.library.body_elements.solid
  Bracket Transform Left : sm_lib/Frames and Transforms/Rigid Transform  TranslationMethod=StandardAxis  TranslationLengthUnit=m  TranslationStandardAxis=+Z  TranslationStandardOffset=(Larm-Warm)/2  TranslationCartesianOffset=[0 0 0]  TranslationROffset=0  TranslationROffsetUnits=m  TranslationZOffset=0  TranslationZOffsetUnits=m  TranslationThetaOffset=0  TranslationThetaOffsetUnits=deg  RotationMethod=AlignedAxes  RotationAngleUnits=deg  RotationStandardAxis=+Y  RotationAngle=180  RotationArbitraryAxis=[0 0 1]  FollAlignAxisA=+Z  BaseAlignAxisA=+Z  FollAlignAxisB=+X  BaseAlignAxisB=+X  BlockFunction=simmechanics.library.frames_transforms.rigid_transform
  Bracket Transform Right : sm_lib/Frames and Transforms/Rigid Transform  TranslationMethod=StandardAxis  TranslationLengthUnit=m  TranslationStandardAxis=-Z  TranslationStandardOffset=(Larm-Warm)/2  TranslationCartesianOffset=[0 0 0]  TranslationROffset=0  TranslationROffsetUnits=m  TranslationZOffset=0  TranslationZOffsetUnits=m  TranslationThetaOffset=0  TranslationThetaOffsetUnits=deg  RotationMethod=AlignedAxes  RotationAngleUnits=deg  RotationStandardAxis=+Y  RotationAngle=180  RotationArbitraryAxis=[0 0 1]  FollAlignAxisA=+Z  BaseAlignAxisA=-Z  FollAlignAxisB=+Y  BaseAlignAxisB=+Y  BlockFunction=simmechanics.library.frames_transforms.rigid_transform
  Bracket Left : Backhoe_Lib/Bracket  Hbracket=Warm  Wbracket=Warm  Tbracket=Tab  Dbracket=Tarm  Hhole=Warm/2  Rhole=RH3  circlePoints=25  bracketColor=hubColor  rho=rho
  Bracket Right : Backhoe_Lib/Bracket  Hbracket=Warm  Wbracket=Warm  Tbracket=Tab  Dbracket=Tarm  Hhole=Warm/2  Rhole=RH3  circlePoints=25  bracketColor=hubColor  rho=rho
  Left Pin : sm_lib/Body Elements/Solid  InertiaType=CalculateFromGeometry  Mass=1  MassUnits=kg  CenterOfMass=[0 0 0]  CenterOfMassUnits=m  MomentsOfInertia=[1 1 1]  MomentsOfInertiaUnits=kg*m^2  ProductsOfInertia=[0 0 0]  ProductsOfInertiaUnits=kg*m^2  DensityBased=on  Density=rhoSteel  DensityUnits=kg/(m^3)  GraphicType=FromGeometry  MarkerShape=Sphere  MarkerSize=10  MarkerSizeUnits=m  GraphicVisPropType=SimpleVisualProperties  GraphicDiffuseColor=gray  GraphicSpecularColor=[0.5 0.5 0.5 1.0]  GraphicAmbientColor=[0.15 0.15 0.15 1.0]  GraphicEmissiveColor=[0.0 0.0 0.0 1.0]  GraphicShininess=75  GraphicOpacity=1.0  GeometryShape=Cylinder  RectangleSize=[1 1]  RectangleSizeUnits=m  BrickDimensions=[3 0.5 0.5]  BrickDimensionUnits=m  CylinderRadius=RH3  CylinderRadiusUnits=m  CylinderLength=Tarm*1.2  CylinderLengthUnits=m  SphereRadius=1  SphereRadiusUnits=m  EllipsoidRadii=[1 1 1]  EllipsoidRadiiUnits=m  ExtrusionCrossSection=[1 1; -1 1; -1 -1; 1 -1]  ExtrusionCrossSectionUnits=m  ExtrusionLength=1  ExtrusionLengthUnits=m  PolygonNumSides=3  PolygonOuterRadius=1  PolygonOuterRadiusUnits=m  ExtGeomFileType=STL  ExtGeomFileUnits=m  RevolutionCrossSection=[1 1; 1 -1; 2 -1; 2 1]  RevolutionCrossSectionUnits=m  RevolutionExtent=Full  RevolutionAngle=180  RevolutionAngleUnits=deg  BlockFunction=simmechanics.library.body_elements.solid
  Plates : Subsystem
      mask Display:
      | image(imread('Backhoe_Mountingplates_IMAGE.png'));
      | port_label('lconn',1,'LA');
      | port_label('lconn',2,'LC');
      | port_label('lconn',3,'AAL');
      | port_label('rconn',1,'B');
      | port_label('rconn',2,'AAR');
  Right Pin : sm_lib/Body Elements/Solid  InertiaType=CalculateFromGeometry  Mass=1  MassUnits=kg  CenterOfMass=[0 0 0]  CenterOfMassUnits=m  MomentsOfInertia=[1 1 1]  MomentsOfInertiaUnits=kg*m^2  ProductsOfInertia=[0 0 0]  ProductsOfInertiaUnits=kg*m^2  DensityBased=on  Density=rhoSteel  DensityUnits=kg/(m^3)  GraphicType=FromGeometry  MarkerShape=Sphere  MarkerSize=10  MarkerSizeUnits=m  GraphicVisPropType=SimpleVisualProperties  GraphicDiffuseColor=gray  GraphicSpecularColor=[0.5 0.5 0.5 1.0]  GraphicAmbientColor=[0.15 0.15 0.15 1.0]  GraphicEmissiveColor=[0.0 0.0 0.0 1.0]  GraphicShininess=75  GraphicOpacity=1.0  GeometryShape=Cylinder  RectangleSize=[1 1]  RectangleSizeUnits=m  BrickDimensions=[3 0.5 0.5]  BrickDimensionUnits=m  CylinderRadius=RH3  CylinderRadiusUnits=m  CylinderLength=Tarm*1.2  CylinderLengthUnits=m  SphereRadius=1  SphereRadiusUnits=m  EllipsoidRadii=[1 1 1]  EllipsoidRadiiUnits=m  ExtrusionCrossSection=[1 1; -1 1; -1 -1; 1 -1]  ExtrusionCrossSectionUnits=m  ExtrusionLength=1  ExtrusionLengthUnits=m  PolygonNumSides=3  PolygonOuterRadius=1  PolygonOuterRadiusUnits=m  ExtGeomFileType=STL  ExtGeomFileUnits=m  RevolutionCrossSection=[1 1; 1 -1; 2 -1; 2 1]  RevolutionCrossSectionUnits=m  RevolutionExtent=Full  RevolutionAngle=180  RevolutionAngleUnits=deg  BlockFunction=simmechanics.library.body_elements.solid
  Single Bracket : Backhoe_Lib/Single Bracket  Hbracket=Lbracket  Wbracket=Dplates-Tplate  Tbracket=Hright  Hhole=Hhole  Rhole=Rhole  Nc=25  bracketColor=orange  rho=rho
  LArm : PMIOPort  Port=1  Side=Right
  LAct : PMIOPort  Port=2  Side=Right
  B : PMIOPort  Port=3  Side=Left
  connections:
  Bracket Transform Right/RConn1 -- Bracket Right/LConn1
  Bracket Right/RConn1 -- Right Pin/RConn1
  Bracket Transform Right/LConn1 -- Plates/RConn2 -- Attachment Arm Right/RConn1
  Bracket Transform Left/RConn1 -- Bracket Left/LConn1
  Left Pin/RConn1 -- Bracket Left/RConn1
  Bracket Transform Left/LConn1 -- Plates/LConn3 -- Attachment Arm Left/RConn1
  Single Bracket/LConn1 -- Plates/RConn1
  Plates/LConn2 -- LAct/RConn1
  Alignment/LConn1 -- B/RConn1
  Alignment/RConn1 -- Single Bracket/RConn1
  Angle Realignment/LConn1 -- Plates/LConn1
  Angle Realignment/RConn1 -- LArm/RConn1

== system Backhoe_Arm/Arm/RotCir  ==
  Rigid Transform1 : sm_lib/Frames and Transforms/Rigid Transform  TranslationMethod=None  TranslationLengthUnit=m  TranslationStandardAxis=+Z  TranslationStandardOffset=0  TranslationCartesianOffset=[0 0 0]  TranslationROffset=0  TranslationROffsetUnits=m  TranslationZOffset=0  TranslationZOffsetUnits=m  TranslationThetaOffset=0  TranslationThetaOffsetUnits=deg  RotationMethod=AlignedAxes  RotationAngleUnits=deg  RotationStandardAxis=+Z  RotationAngle=0  RotationArbitraryAxis=[0 0 1]  FollAlignAxisA=+X  BaseAlignAxisA=+Z  FollAlignAxisB=+Y  BaseAlignAxisB=+Y  BlockFunction=simmechanics.library.frames_transforms.rigid_transform
  RotCir : Subsystem  mask{W=1, T=0.15, R=0.075, Rho=2700, LinkRGB=[0.8396    0.5433         0]}
      mask init:
      | % Cross-section of Main:
      | Alpha = (pi/2:-0.01:-pi/2)';
      | Beta = (3*pi/2:-0.01:pi/2)';
      | 
      | % Cross-section of HoleA:
      | Alpha = (pi/2:0.01:3*pi/2)';
      | Beta = (3*pi/2:-0.01:pi/2)';
      | HoleACS = [W/2*cos(Alpha) W/2*sin(Alpha);...
      | R*cos(Beta) R*sin(Beta)];
      | 
      | % Cross-section of HoleB:
      | Alpha = (-pi/2:0.01:pi/2)';
      | Beta = (pi/2:-0.01:-pi/2)';
      | HoleBCS = [W/2*cos(Alpha) W/2*sin(Alpha);...
      | R*cos(Beta) R*sin(Beta)];
  Conn1 : PMIOPort  Port=1  Side=Left
  Conn2 : PMIOPort  Port=2  Side=Right
  connections:
  Conn1/RConn1 -- RotCir/LConn1
  Rigid Transform1/RConn1 -- Conn2/RConn1
  RotCir/RConn1 -- Rigid Transform1/LConn1

== system Backhoe_Arm/Arm/RotCir1 ==
  Rigid Transform2 : sm_lib/Frames and Transforms/Rigid Transform  TranslationMethod=None  TranslationLengthUnit=m  TranslationStandardAxis=+Z  TranslationStandardOffset=0  TranslationCartesianOffset=[0 0 0]  TranslationROffset=0  TranslationROffsetUnits=m  TranslationZOffset=0  TranslationZOffsetUnits=m  TranslationThetaOffset=0  TranslationThetaOffsetUnits=deg  RotationMethod=AlignedAxes  RotationAngleUnits=deg  RotationStandardAxis=+Z  RotationAngle=0  RotationArbitraryAxis=[0 0 1]  FollAlignAxisA=+X  BaseAlignAxisA=+Z  FollAlignAxisB=+Y  BaseAlignAxisB=+Y  BlockFunction=simmechanics.library.frames_transforms.rigid_transform
  RotCir2 : Subsystem  mask{W=1, T=0.15, R=0.075, Rho=2700, LinkRGB=[0.8396    0.5433         0]}
      mask init: same as Backhoe_Arm/Arm/RotCir /RotCir
  Conn1 : PMIOPort  Port=1  Side=Left
  Conn2 : PMIOPort  Port=2  Side=Right
  connections:
  Conn1/RConn1 -- RotCir2/LConn1
  RotCir2/RConn1 -- Rigid Transform2/LConn1
  Rigid Transform2/RConn1 -- Conn2/RConn1
